simulink model "Acc_Dec"  (R2024a)
settings: Solver=VariableStepAuto  StartTime=0.0  StopTime=10.0  RelTol=1e-3
libraries: simulink x3
settings Model: Creator=User  LastModifiedBy=User

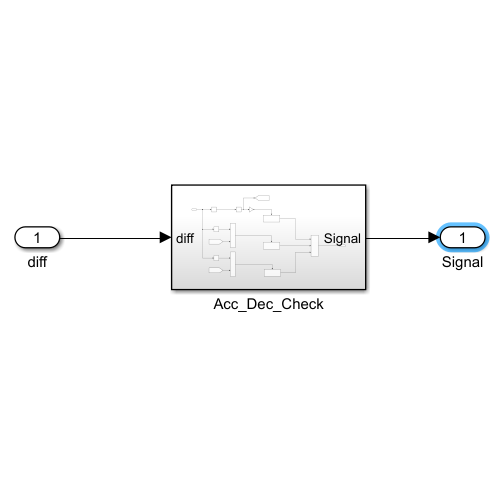
[thumbnail: Simulink's stored preview of the top-level diagram]
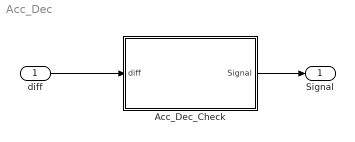
== system Acc_Dec ==
  diff : Inport
  Acc_Dec_Check : Subsystem
  Signal : Outport
  wires:
  diff/1 -> Acc_Dec_Check/1(diff)
  Acc_Dec_Check/1(Signal) -> Signal/1

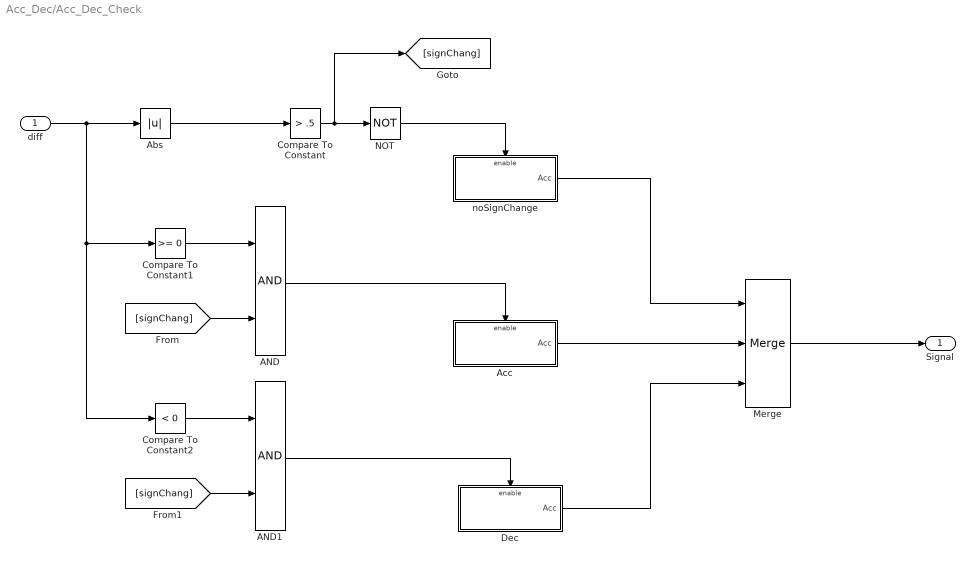
== system Acc_Dec/Acc_Dec_Check ==
  diff : Inport
  AND : Logic  AllPortsSameDT=off  OutDataTypeStr=boolean
  AND1 : Logic  AllPortsSameDT=off  OutDataTypeStr=boolean
  Abs : Abs  SaturateOnIntegerOverflow=off
  Acc : Subsystem  TreatAsAtomicUnit=on
  Compare To Constant : simulink/Logic and Bit Operations/Compare To Constant  relop=>  const=.5  OutDataTypeStr=boolean
  Compare To Constant1 : simulink/Logic and Bit Operations/Compare To Constant  relop=>=  const=0  OutDataTypeStr=boolean
  Compare To Constant2 : simulink/Logic and Bit Operations/Compare To Constant  relop=<  const=0  OutDataTypeStr=boolean
  Dec : Subsystem  TreatAsAtomicUnit=on
  Merge : Merge  Inputs=3
  NOT : Logic  Operator=NOT  IconShape=distinctive  AllPortsSameDT=off  OutDataTypeStr=boolean
  noSignChange : Subsystem  TreatAsAtomicUnit=on
  Signal : Outport
  wires:
  Merge/1 -> Signal/1
  Compare To Constant/1 -> [signChang], NOT/1
  Compare To Constant1/1 -> AND/1
  noSignChange/1(Acc) -> Merge/1
  diff/1 -> Compare To Constant2/1, Compare To Constant1/1, Abs/1
  Abs/1 -> Compare To Constant/1
  NOT/1 -> noSignChange/Enable
  AND/1 -> Acc/Enable
  [signChang] -> AND/2
  AND1/1 -> Dec/Enable
  Acc/1(Acc) -> Merge/2
  [signChang] -> AND1/2
  Dec/1(Acc) -> Merge/3
  Compare To Constant2/1 -> AND1/1

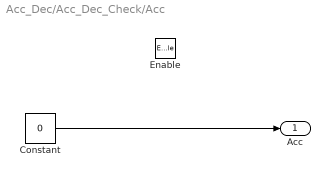
== system Acc_Dec/Acc_Dec_Check/Acc ==
  Enable : EnablePort
  Constant : Constant  Value=0
  Acc : Outport
  wires:
  Constant/1 -> Acc/1

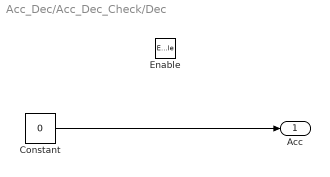
== system Acc_Dec/Acc_Dec_Check/Dec ==
  Enable : EnablePort
  Constant : Constant  Value=0
  Acc : Outport
  wires:
  Constant/1 -> Acc/1

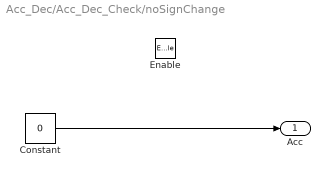
== system Acc_Dec/Acc_Dec_Check/noSignChange ==
  Enable : EnablePort
  Constant : Constant  Value=0
  Acc : Outport
  wires:
  Constant/1 -> Acc/1
